simulink model "task10"  (R2023a)
settings: Solver=ode15s  StartTime=0.0  StopTime=10.0  RelTol=1e-3
undefined symbols (not defined in the file or in its folder): DisplayTrajectoryImpedance
settings Model: Creator=LENOVO  LastModifiedBy=LENOVO

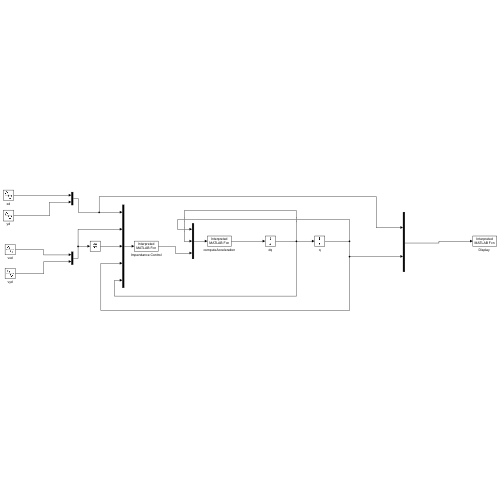
[thumbnail: Simulink's stored preview of the top-level diagram]
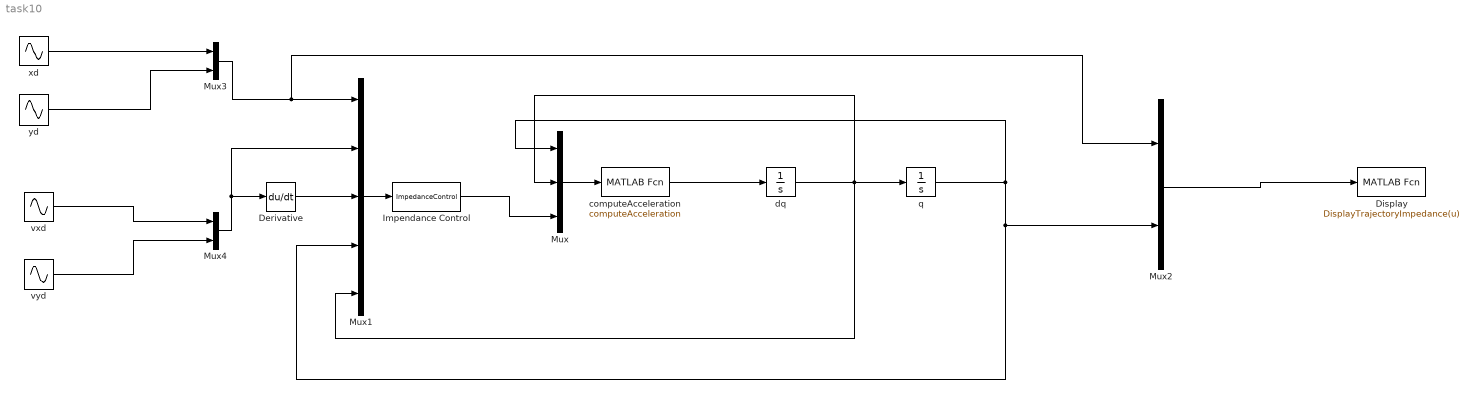
== system task10 ==
  Derivative : Derivative
  "Display " : MATLABFcn  MATLABFcn=DisplayTrajectoryImpedance(u)  OutputDimensions=0
  Impendance Control : MATLABFcn  MATLABFcn=ImpedanceControl  OutputDimensions=2
  Mux : Mux  Inputs=3
  Mux1 : Mux  Inputs=5
  Mux2 : Mux  Inputs=2
  Mux3 : Mux  Inputs=2
  Mux4 : Mux  Inputs=2
  computeAcceleration : MATLABFcn  MATLABFcn=computeAcceleration  OutputDimensions=2  Output1D=off
  dq : Integrator  InitialCondition=[0; 0]
  q : Integrator  InitialCondition=[pi/2; pi/4]
  vxd : Sin  Amplitude=0.1*2/3*pi  Frequency=0.8*2*pi  Phase=90  SampleTime=0
  vyd : Sin  Amplitude=0.3*2/3*pi  Frequency=2*0.8*pi  Phase=90  SampleTime=0
  xd : Sin  Amplitude=0.1  Bias=0.2  Frequency=0.8*2*pi  SampleTime=0
  yd : Sin  Amplitude=0.3  Bias=0.2  Frequency=0.8*2*pi  SampleTime=0
  wires:
  Mux2/1 -> "Display "/1
  Impendance Control/1 -> Mux/3
  Mux1/1 -> Impendance Control/1
  dq/1 -> Mux1/5, Mux/2, q/1
  computeAcceleration/1 -> dq/1
  q/1 -> Mux1/4, Mux2/2, Mux/1
  Mux/1 -> computeAcceleration/1
  vxd/1 -> Mux4/1
  xd/1 -> Mux3/1
  vyd/1 -> Mux4/2
  yd/1 -> Mux3/2
  Mux3/1 -> Mux2/1, Mux1/1
  Mux4/1 -> Derivative/1, Mux1/2
  Derivative/1 -> Mux1/3
